simulink subsystem "FreqSweep"  (R2025a)
settings: Solver=VariableStepAuto  StartTime=0.0  StopTime=10.0  RelTol=1e-3
settings Model: Creator=17036  LastModifiedBy=gurt1

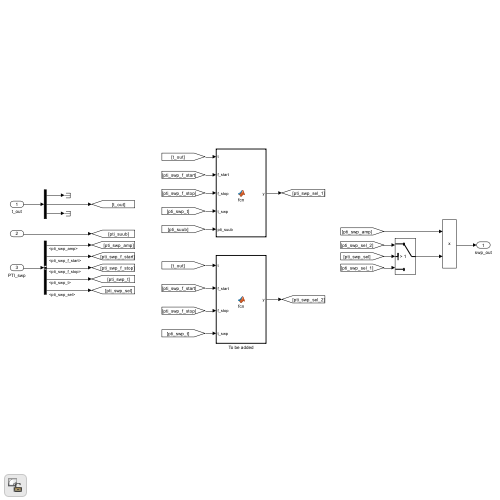
[thumbnail: Simulink's stored preview of the top-level diagram]
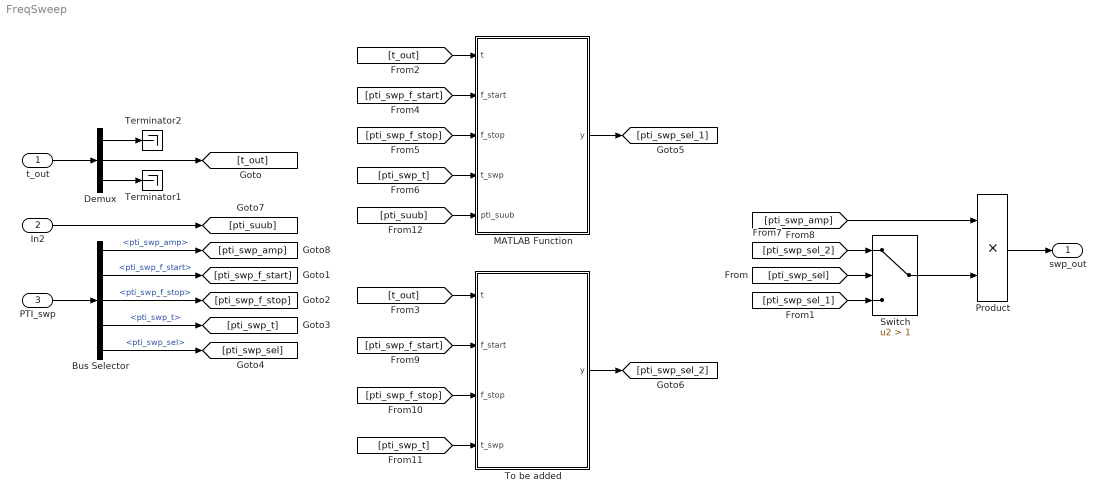
== system FreqSweep ==
  t_out : Inport
  In2 : Inport  Port=2
  PTI_swp : Inport  Port=3
  Bus Selector : BusSelector  OutputSignals=pti_swp_amp,pti_swp_f_start,pti_swp_f_stop,pti_swp_t,pti_swp_sel
  Demux : Demux  Outputs=3
  MATLAB Function : MATLAB Function  TreatAsAtomicUnit=on
  Product : Product
  Switch : Switch  Criteria=u2 > Threshold  Threshold=1  SaturateOnIntegerOverflow=off  InputSameDT=off
  Terminator1 : Terminator
  Terminator2 : Terminator
  To be added : MATLAB Function  TreatAsAtomicUnit=on
  swp_out : Outport
  wires:
  PTI_swp/1 -> Bus Selector/1
  Bus Selector/1 -> [pti_swp_amp]  "<pti_swp_amp>"
  Bus Selector/2 -> [pti_swp_f_start]  "<pti_swp_f_start>"
  Bus Selector/3 -> [pti_swp_f_stop]  "<pti_swp_f_stop>"
  Bus Selector/4 -> [pti_swp_t]  "<pti_swp_t>"
  Bus Selector/5 -> [pti_swp_sel]  "<pti_swp_sel>"
  [pti_swp_sel] -> Switch/2
  MATLAB Function/1(y) -> [pti_swp_sel_1]
  [t_out] -> MATLAB Function/1(t)
  [pti_swp_f_start] -> MATLAB Function/2(f_start)
  [pti_swp_f_stop] -> MATLAB Function/3(f_stop)
  [pti_swp_t] -> MATLAB Function/4(t_swp)
  Switch/1 -> Product/2
  [pti_swp_amp] -> Product/1
  Product/1 -> swp_out/1
  t_out/1 -> Demux/1
  Demux/3 -> Terminator1/1
  [t_out] -> To be added/1(t)
  [pti_swp_t] -> To be added/4(t_swp)
  [pti_swp_f_stop] -> To be added/3(f_stop)
  To be added/1(y) -> [pti_swp_sel_2]
  [pti_swp_f_start] -> To be added/2(f_start)
  Demux/2 -> [t_out]
  Demux/1 -> Terminator2/1
  [pti_swp_sel_2] -> Switch/1
  [pti_swp_sel_1] -> Switch/3
  In2/1 -> [pti_suub]
  [pti_suub] -> MATLAB Function/5(pti_suub)

== matlab function FreqSweep/MATLAB Function ==
  data: t input; y output; f_start input; f_stop input; t_swp input; pti_suub input
function y = fcn(t,f_start,f_stop,t_swp, pti_suub)

% Mixing matrix for quadcopter control (roll, pitch, yaw, throttle)
M = [-1  1 -1 1;
      1 -1 -1 1;
      1  1  1 1;
     -1 -1  1 1];

% Select the column corresponding to the axis mode
axis_mode = M(:,pti_suub+1);

if t<=t_swp
    % Calculate instantaneous frequency
    f_inst = (f_stop-f_start)*t/t_swp+f_start;
    
    % Generate sinusoidal signal with the calculated frequency
    swp = sin(2*pi*f_inst*t);
else
    swp = 0;
end

y = swp.*axis_mode;

== matlab function FreqSweep/To be added ==
  data: t input; y output; f_start input; f_stop input; t_swp input
function y = fcn(t,f_start,f_stop,t_swp)

if t<=t_swp
    % Calculate instantaneous frequency
    f_inst = (f_stop-f_start)*t/t_swp+f_start;
    
    % Generate sinusoidal signal with the calculated frequency
    y = sin(2*pi*f_inst*t);
else
    y = 0;
end
